simulink library "funcsetup"  (Simulink 5.0)
values from neighbouring files (symbols this model uses):
  RndMeth = 'floor'    [fixpt_interp1.m]
undefined symbols (not defined in the file or in its folder): ErrMax, ErrMax_nonvisible, Nptsmax, Nptsmax_nonvisible, RndMeth_nonvisible, Spacing, Spacing_nonvisible, xData, xData_nonvisible, xDt, xDt_nonvisible, xmax, xMax_nonvisible, xmin, xMin_nonvisible, xScale, xScale_nonvisible, yData, yData_nonvisible, yDt, yDt_nonvisible, yScale, yScale_nonvisible
settings Model: Creator=krishnan  LastModifiedBy=krishnan  ExtModeAutoUpdateStatusClock=off

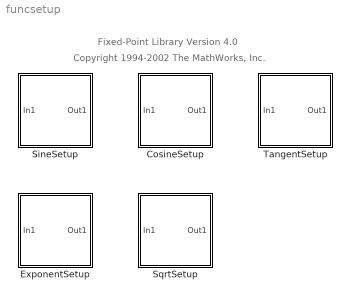
== system funcsetup ==
  note: Fixed-Point Library Version 4.0
  note: Copyright 1994-2002 The MathWorks, Inc.
  CosineSetup : Subsystem  mask(MEGMA CosineSetup){yData=yData, xData=xData, yData_nonvisible=yData_nonvisible, xData_nonvisible=xData_nonvisible, Spacing_nonvisible=Spacing_nonvisible, Nptsmax_nonvisible=Nptsmax_nonvisible, ErrMax_nonvisible=ErrMax_nonvisible, RndMeth_nonvisible=RndMeth_nonvisible, yScale_nonvisible=yScale_nonvisible, yDt_nonvisible=yDt_nonvisible, xScale_nonvisible=xScale_nonvisible, xDt_nonvisible=xDt_nonvisible, xMax_nonvisible=xMax_nonvisible, xMin_nonvisible=xMin_nonvisible, Spacing=Spacing, Nptsmax=Nptsmax, ErrMax=ErrMax, RndMeth=RndMeth, yScale=yScale, xScale=xScale, yDt=yDt, xDt=xDt, xmax=xmax, xmin=xmin}
      mask prompts: Spacing "Allowed spacing 'pow2','even', or 'unrestricted'(default)"; Nptsmax "Maximum number of breakpoints"; ErrMax "Maximum worst case approximation error"; RndMeth "Rounding method 'floor'(default),'ceil','near' or 'zero'"; yScale "Output Scaling"; xScale "Input Scaling"; yDt "Output Datatype"; xDt "Input Datatype"; xmax "Maximum input value of interest"; xmin "Minimum input value of interest"
      mask help: MEGMA CosineSetup
      mask init:
      | FuncStr = 'cos(x)';
      |  par = get_param(gcb,'parent');
      | Recompute = get_param(par,'Recompute');
      | if strcmp(Recompute,'Cache across different MATLAB sessions')
      | Recompute = 3;
      | end
      | if Recompute == 3
      |   if ~isequal(Spacing, Spacing_nonvisible) | ~isequal(Nptsmax,Nptsmax_nonvisible) ...
      | 	|~isequal(ErrMax,ErrMax_nonvisible) | ~isequal(xmin,xMin_nonvisible) ...
      | 	| ~isequal(xmax,xMax_nonvisible) | ~isequal(xDt,xDt_nonvisible) | ...
      | 	~isequal(xScale,xScale_nonvisible) | ~isequal(yDt,yDt_nonvisible) | ...
      | 	~isequal(yScale,yScale_nonvisible) | ~isequal(RndMeth,RndMeth_nonvisible) ...
      | 	| ~isequal(xData,xData_nonvisible) | ~isequal(yData,yData_nonvisible)
      |     text_new_Spacing = get_param(par,'Spacing');
      |     text_new_Nptsmax = get_param(par,'Nptsmax');
      |     text_new_ErrMax  = get_param(par,'ErrMax');
      |     text_new_xmin    = get_param(par,'xmin');
      |     text_new_xmax    = get_param(par,'xmax');
      |     text_new_xDt     = get_param(par,'xDt');
      |     text_new_xScale  = get_param(par,'xScale');
      |     text_new_yDt     = get_param(par,'yDt');
      |     text_new_yScale  = get_param(par,'yScale');
      |     text_new_RndMeth = get_param(par,'RndMeth');
      |     set_param(par,'Spacing_nonvisible',text_new_Spacing);
      |     set_param(par,'Nptsmax_nonvisible',text_new_Nptsmax);
      |     set_param(par,'ErrMax_nonvisible',text_new_ErrMax);
      |     set_param(par,'xMin_nonvisible',text_new_xmin);
      |     set_param(par,'xMax_nonvisible',text_new_xmax);
      |     set_param(par,'xDt_nonvisible',text_new_xDt);
      |     set_param(par,'xScale_nonvisible',text_new_xScale);
      |     set_param(par,'yDt_nonvisible',text_new_yDt);
      |     set_param(par,'yScale_nonvisible',text_new_yScale);
      |     set_param(par,'RndMeth_nonvisible',text_new_RndMeth);
      |     [xData,yData]= fixpt_look1_func_approx(FuncStr,xmin,xmax,xDt,xScale,yDt, ...
      | 					   yScale,RndMeth,...
      | 					   ErrMax,Nptsmax,Spacing,Recompute);
      |     set_param(par,'xData',mat2str(xData));
      |     set_param(par,'yData',mat2str(yData));
      |     set_param(par,'xData_nonvisible',mat2str(xData));
      |     set_param(par,'yData_nonvisible',mat2str(yData));
      |   end
      | end
      mask Help: web(fpbhelp('cosinesetup'));
      mask Display:
      | disp('CosineSetup')
      | patch([2 2 10 10 4 4 8 8 4 4 2 ],[2 10 10 8 8 6 6 4 4 2 2 ],[0 0 0],'bottom-right');
  ExponentSetup : Subsystem  mask(MEGMA ExponentSetup){yData=yData, xData=xData, yData_nonvisible=yData_nonvisible, xData_nonvisible=xData_nonvisible, Spacing_nonvisible=Spacing_nonvisible, Nptsmax_nonvisible=Nptsmax_nonvisible, ErrMax_nonvisible=ErrMax_nonvisible, RndMeth_nonvisible=RndMeth_nonvisible, yScale_nonvisible=yScale_nonvisible, yDt_nonvisible=yDt_nonvisible, xScale_nonvisible=xScale_nonvisible, xDt_nonvisible=xDt_nonvisible, xMax_nonvisible=xMax_nonvisible, xMin_nonvisible=xMin_nonvisible, Spacing=Spacing, Nptsmax=Nptsmax, ErrMax=ErrMax, RndMeth=RndMeth, yScale=yScale, xScale=xScale, yDt=yDt, xDt=xDt, xmax=xmax, xmin=xmin}
      mask prompts: Spacing "Allowed spacing 'pow2','even', or 'unrestricted'(default)"; Nptsmax "Maximum number of breakpoints"; ErrMax "Maximum worst case approximation error"; RndMeth "Rounding method 'floor'(default),'ceil','near' or 'zero'"; yScale "Output Scaling"; xScale "Input Scaling"; yDt "Output Datatype"; xDt "Input Datatype"; xmax "Maximum input value of interest"; xmin "Minimum input value of interest"
      mask help: MEGMA ExponentSetup
      mask init:
      | FuncStr = 'exp(x)';
      |  par = get_param(gcb,'parent');
      | Recompute = get_param(par,'Recompute');
      | if strcmp(Recompute,'Cache across different MATLAB sessions')
      | Recompute = 3;
      | end
      | if Recompute == 3
      |   if ~isequal(Spacing, Spacing_nonvisible) | ~isequal(Nptsmax,Nptsmax_nonvisible) ...
      | 	|~isequal(ErrMax,ErrMax_nonvisible) | ~isequal(xmin,xMin_nonvisible) ...
      | 	| ~isequal(xmax,xMax_nonvisible) | ~isequal(xDt,xDt_nonvisible) | ...
      | 	~isequal(xScale,xScale_nonvisible) | ~isequal(yDt,yDt_nonvisible) | ...
      | 	~isequal(yScale,yScale_nonvisible) | ~isequal(RndMeth,RndMeth_nonvisible) ...
      | 	| ~isequal(xData,xData_nonvisible) | ~isequal(yData,yData_nonvisible)
      |     text_new_Spacing = get_param(par,'Spacing');
      |     text_new_Nptsmax = get_param(par,'Nptsmax');
      |     text_new_ErrMax  = get_param(par,'ErrMax');
      |     text_new_xmin    = get_param(par,'xmin');
      |     text_new_xmax    = get_param(par,'xmax');
      |     text_new_xDt     = get_param(par,'xDt');
      |     text_new_xScale  = get_param(par,'xScale');
      |     text_new_yDt     = get_param(par,'yDt');
      |     text_new_yScale  = get_param(par,'yScale');
      |     text_new_RndMeth = get_param(par,'RndMeth');
      |     set_param(par,'Spacing_nonvisible',text_new_Spacing);
      |     set_param(par,'Nptsmax_nonvisible',text_new_Nptsmax);
      |     set_param(par,'ErrMax_nonvisible',text_new_ErrMax);
      |     set_param(par,'xMin_nonvisible',text_new_xmin);
      |     set_param(par,'xMax_nonvisible',text_new_xmax);
      |     set_param(par,'xDt_nonvisible',text_new_xDt);
      |     set_param(par,'xScale_nonvisible',text_new_xScale);
      |     set_param(par,'yDt_nonvisible',text_new_yDt);
      |     set_param(par,'yScale_nonvisible',text_new_yScale);
      |     set_param(par,'RndMeth_nonvisible',text_new_RndMeth);
      |     [xData,yData]= fixpt_look1_func_approx(FuncStr,xmin,xmax,xDt,xScale,yDt, ...
      | 					   yScale,RndMeth,...
      | 					   ErrMax,Nptsmax,Spacing,Recompute);
      |     set_param(par,'xData',mat2str(xData));
      |     set_param(par,'yData',mat2str(yData));
      |     set_param(par,'xData_nonvisible',mat2str(xData));
      |     set_param(par,'yData_nonvisible',mat2str(yData));
      |   end
      | end
      mask Help: web(fpbhelp('exponentsetup'));
      mask Display:
      | disp('ExponentSetup')
      | patch([2 2 10 10 4 4 8 8 4 4 2 ],[2 10 10 8 8 6 6 4 4 2 2 ],[0 0 0],'bottom-right');
  SineSetup : Subsystem  mask(MEGMA SineSetup){yData=yData, xData=xData, yData_nonvisible=yData_nonvisible, xData_nonvisible=xData_nonvisible, Spacing_nonvisible=Spacing_nonvisible, Nptsmax_nonvisible=Nptsmax_nonvisible, ErrMax_nonvisible=ErrMax_nonvisible, RndMeth_nonvisible=RndMeth_nonvisible, yScale_nonvisible=yScale_nonvisible, yDt_nonvisible=yDt_nonvisible, xScale_nonvisible=xScale_nonvisible, xDt_nonvisible=xDt_nonvisible, xMax_nonvisible=xMax_nonvisible, xMin_nonvisible=xMin_nonvisible, Spacing=Spacing, Nptsmax=Nptsmax, ErrMax=ErrMax, RndMeth=RndMeth, yScale=yScale, xScale=xScale, yDt=yDt, xDt=xDt, xmax=xmax, xmin=xmin}
      mask prompts: Spacing "Allowed spacing 'pow2','even', or 'unrestricted'(default)"; Nptsmax "Maximum number of breakpoints"; ErrMax "Maximum worst case approximation error"; RndMeth "Rounding method 'floor'(default),'ceil','near' or 'zero'"; yScale "Output Scaling"; xScale "Input Scaling"; yDt "Output Datatype"; xDt "Input Datatype"; xmax "Maximum input value of interest"; xmin "Minimum input value of interest"
      mask help: MEGMA SineSetup
      mask init:
      | FuncStr = 'sin(x)';
      |  par = get_param(gcb,'parent');
      | Recompute  = get_param(par,'Recompute');
      | if strcmp(Recompute,'Cache across different MATLAB sessions')
      | Recompute = 3;
      | end
      | if Recompute == 3
      |   if ~isequal(Spacing, Spacing_nonvisible) | ~isequal(Nptsmax,Nptsmax_nonvisible) ...
      | 	|~isequal(ErrMax,ErrMax_nonvisible) | ~isequal(xmin,xMin_nonvisible) ...
      | 	| ~isequal(xmax,xMax_nonvisible) | ~isequal(xDt,xDt_nonvisible) | ...
      | 	~isequal(xScale,xScale_nonvisible) | ~isequal(yDt,yDt_nonvisible) | ...
      | 	~isequal(yScale,yScale_nonvisible) | ~isequal(RndMeth,RndMeth_nonvisible) ...
      | 	| ~isequal(xData,xData_nonvisible) | ~isequal(yData,yData_nonvisible)
      |     text_new_Spacing = get_param(par,'Spacing');
      |     text_new_Nptsmax = get_param(par,'Nptsmax');
      |     text_new_ErrMax  = get_param(par,'ErrMax');
      |     text_new_xmin    = get_param(par,'xmin');
      |     text_new_xmax    = get_param(par,'xmax');
      |     text_new_xDt     = get_param(par,'xDt');
      |     text_new_xScale  = get_param(par,'xScale');
      |     text_new_yDt     = get_param(par,'yDt');
      |     text_new_yScale  = get_param(par,'yScale');
      |     text_new_RndMeth = get_param(par,'RndMeth');
      |     set_param(par,'Spacing_nonvisible',text_new_Spacing);
      |     set_param(par,'Nptsmax_nonvisible',text_new_Nptsmax);
      |     set_param(par,'ErrMax_nonvisible',text_new_ErrMax);
      |     set_param(par,'xMin_nonvisible',text_new_xmin);
      |     set_param(par,'xMax_nonvisible',text_new_xmax);
      |     set_param(par,'xDt_nonvisible',text_new_xDt);
      |     set_param(par,'xScale_nonvisible',text_new_xScale);
      |     set_param(par,'yDt_nonvisible',text_new_yDt);
      |     set_param(par,'yScale_nonvisible',text_new_yScale);
      |     set_param(par,'RndMeth_nonvisible',text_new_RndMeth);
      |     [xData,yData]= fixpt_look1_func_approx(FuncStr,xmin,xmax,xDt,xScale,yDt, ...
      | 					   yScale,RndMeth,...
      | 					   ErrMax,Nptsmax,Spacing,Recompute);
      |     set_param(par,'xData',mat2str(xData));
      |     set_param(par,'yData',mat2str(yData));
      |     set_param(par,'xData_nonvisible',mat2str(xData));
      |     set_param(par,'yData_nonvisible',mat2str(yData));
      |   end
      | end
      mask Help: web(fpbhelp('sinesetup'));
      mask Display:
      | disp('SineSetup')
      | patch([2 2 10 10 4 4 8 8 4 4 2 ],[2 10 10 8 8 6 6 4 4 2 2 ],[0 0 0],'bottom-right');
  SqrtSetup : Subsystem  mask(MEGMA SqrtSetup){yData=yData, xData=xData, yData_nonvisible=yData_nonvisible, xData_nonvisible=xData_nonvisible, Spacing_nonvisible=Spacing_nonvisible, Nptsmax_nonvisible=Nptsmax_nonvisible, ErrMax_nonvisible=ErrMax_nonvisible, RndMeth_nonvisible=RndMeth_nonvisible, yScale_nonvisible=yScale_nonvisible, yDt_nonvisible=yDt_nonvisible, xScale_nonvisible=xScale_nonvisible, xDt_nonvisible=xDt_nonvisible, xMax_nonvisible=xMax_nonvisible, xMin_nonvisible=xMin_nonvisible, Spacing=Spacing, Nptsmax=Nptsmax, ErrMax=ErrMax, RndMeth=RndMeth, yScale=yScale, xScale=xScale, yDt=yDt, xDt=xDt, xmax=xmax, xmin=xmin}
      mask prompts: Spacing "Allowed spacing 'pow2','even', or 'unrestricted'(default)"; Nptsmax "Maximum number of breakpoints"; ErrMax "Maximum worst case approximation error"; RndMeth "Rounding method 'floor'(default),'ceil','near' or 'zero'"; yScale "Output Scaling"; xScale "Input Scaling"; yDt "Output Datatype"; xDt "Input Datatype"; xmax "Maximum input value of interest"; xmin "Minimum input value of interest"
      mask help: MEGMA SqrtSetup
      mask init:
      | FuncStr = 'sqrt(x)';
      |  par = get_param(gcb,'parent');
      | Recompute = get_param(par,'Recompute');
      | if strcmp(Recompute,'Cache across different MATLAB sessions')
      | Recompute = 3;
      | end
      | if Recompute == 3
      |   if ~isequal(Spacing, Spacing_nonvisible) | ~isequal(Nptsmax,Nptsmax_nonvisible) ...
      | 	|~isequal(ErrMax,ErrMax_nonvisible) | ~isequal(xmin,xMin_nonvisible) ...
      | 	| ~isequal(xmax,xMax_nonvisible) | ~isequal(xDt,xDt_nonvisible) | ...
      | 	~isequal(xScale,xScale_nonvisible) | ~isequal(yDt,yDt_nonvisible) | ...
      | 	~isequal(yScale,yScale_nonvisible) | ~isequal(RndMeth,RndMeth_nonvisible) ...
      | 	| ~isequal(xData,xData_nonvisible) | ~isequal(yData,yData_nonvisible)
      |     text_new_Spacing = get_param(par,'Spacing');
      |     text_new_Nptsmax = get_param(par,'Nptsmax');
      |     text_new_ErrMax  = get_param(par,'ErrMax');
      |     text_new_xmin    = get_param(par,'xmin');
      |     text_new_xmax    = get_param(par,'xmax');
      |     text_new_xDt     = get_param(par,'xDt');
      |     text_new_xScale  = get_param(par,'xScale');
      |     text_new_yDt     = get_param(par,'yDt');
      |     text_new_yScale  = get_param(par,'yScale');
      |     text_new_RndMeth = get_param(par,'RndMeth');
      |     set_param(par,'Spacing_nonvisible',text_new_Spacing);
      |     set_param(par,'Nptsmax_nonvisible',text_new_Nptsmax);
      |     set_param(par,'ErrMax_nonvisible',text_new_ErrMax);
      |     set_param(par,'xMin_nonvisible',text_new_xmin);
      |     set_param(par,'xMax_nonvisible',text_new_xmax);
      |     set_param(par,'xDt_nonvisible',text_new_xDt);
      |     set_param(par,'xScale_nonvisible',text_new_xScale);
      |     set_param(par,'yDt_nonvisible',text_new_yDt);
      |     set_param(par,'yScale_nonvisible',text_new_yScale);
      |     set_param(par,'RndMeth_nonvisible',text_new_RndMeth);
      |     [xData,yData]= fixpt_look1_func_approx(FuncStr,xmin,xmax,xDt,xScale,yDt, ...
      | 					   yScale,RndMeth,...
      | 					   ErrMax,Nptsmax,Spacing,Recompute);
      |     set_param(par,'xData',mat2str(xData));
      |     set_param(par,'yData',mat2str(yData));
      |     set_param(par,'xData_nonvisible',mat2str(xData));
      |     set_param(par,'yData_nonvisible',mat2str(yData));
      |   end
      | end
      mask Help: web(fpbhelp('sqrtsetup'));
      mask Display:
      | disp('SqrtSetup')
      | patch([2 2 10 10 4 4 8 8 4 4 2 ],[2 10 10 8 8 6 6 4 4 2 2 ],[0 0 0],'bottom-right');
  TangentSetup : Subsystem  mask(MEGMA TangentSetup){yData=yData, xData=xData, yData_nonvisible=yData_nonvisible, xData_nonvisible=xData_nonvisible, Spacing_nonvisible=Spacing_nonvisible, Nptsmax_nonvisible=Nptsmax_nonvisible, ErrMax_nonvisible=ErrMax_nonvisible, RndMeth_nonvisible=RndMeth_nonvisible, yScale_nonvisible=yScale_nonvisible, yDt_nonvisible=yDt_nonvisible, xScale_nonvisible=xScale_nonvisible, xDt_nonvisible=xDt_nonvisible, xMax_nonvisible=xMax_nonvisible, xMin_nonvisible=xMin_nonvisible, Spacing=Spacing, Nptsmax=Nptsmax, ErrMax=ErrMax, RndMeth=RndMeth, yScale=yScale, xScale=xScale, yDt=yDt, xDt=xDt, xmax=xmax, xmin=xmin}
      mask prompts: Spacing "Allowed spacing 'pow2','even', or 'unrestricted'(default)"; Nptsmax "Maximum number of breakpoints"; ErrMax "Maximum worst case approximation error"; RndMeth "Rounding method 'floor'(default),'ceil','near' or 'zero'"; yScale "Output Scaling"; xScale "Input Scaling"; yDt "Output Datatype"; xDt "Input Datatype"; xmax "Maximum input value of interest"; xmin "Minimum input value of interest"
      mask help: MEGMA TangentSetup
      mask init:
      | FuncStr = 'tan(x)';
      |  par = get_param(gcb,'parent');
      | Recompute = get_param(par,'Recompute');
      | if strcmp(Recompute,'Cache across different MATLAB sessions')
      | Recompute = 3;
      | end
      | if Recompute == 3
      |   if ~isequal(Spacing, Spacing_nonvisible) | ~isequal(Nptsmax,Nptsmax_nonvisible) ...
      | 	|~isequal(ErrMax,ErrMax_nonvisible) | ~isequal(xmin,xMin_nonvisible) ...
      | 	| ~isequal(xmax,xMax_nonvisible) | ~isequal(xDt,xDt_nonvisible) | ...
      | 	~isequal(xScale,xScale_nonvisible) | ~isequal(yDt,yDt_nonvisible) | ...
      | 	~isequal(yScale,yScale_nonvisible) | ~isequal(RndMeth,RndMeth_nonvisible) ...
      | 	| ~isequal(xData,xData_nonvisible) | ~isequal(yData,yData_nonvisible)
      |     text_new_Spacing = get_param(par,'Spacing');
      |     text_new_Nptsmax = get_param(par,'Nptsmax');
      |     text_new_ErrMax  = get_param(par,'ErrMax');
      |     text_new_xmin    = get_param(par,'xmin');
      |     text_new_xmax    = get_param(par,'xmax');
      |     text_new_xDt     = get_param(par,'xDt');
      |     text_new_xScale  = get_param(par,'xScale');
      |     text_new_yDt     = get_param(par,'yDt');
      |     text_new_yScale  = get_param(par,'yScale');
      |     text_new_RndMeth = get_param(par,'RndMeth');
      |     set_param(par,'Spacing_nonvisible',text_new_Spacing);
      |     set_param(par,'Nptsmax_nonvisible',text_new_Nptsmax);
      |     set_param(par,'ErrMax_nonvisible',text_new_ErrMax);
      |     set_param(par,'xMin_nonvisible',text_new_xmin);
      |     set_param(par,'xMax_nonvisible',text_new_xmax);
      |     set_param(par,'xDt_nonvisible',text_new_xDt);
      |     set_param(par,'xScale_nonvisible',text_new_xScale);
      |     set_param(par,'yDt_nonvisible',text_new_yDt);
      |     set_param(par,'yScale_nonvisible',text_new_yScale);
      |     set_param(par,'RndMeth_nonvisible',text_new_RndMeth);
      |     [xData,yData]= fixpt_look1_func_approx(FuncStr,xmin,xmax,xDt,xScale,yDt, ...
      | 					   yScale,RndMeth,...
      | 					   ErrMax,Nptsmax,Spacing,Recompute);
      |     set_param(par,'xData',mat2str(xData));
      |     set_param(par,'yData',mat2str(yData));
      |     set_param(par,'xData_nonvisible',mat2str(xData));
      |     set_param(par,'yData_nonvisible',mat2str(yData));
      |   end
      | end
      mask Help: web(fpbhelp('tangentsetup'));
      mask Display:
      | disp('TangentSetup')
      | patch([2 2 10 10 4 4 8 8 4 4 2 ],[2 10 10 8 8 6 6 4 4 2 2 ],[0 0 0],'bottom-right');

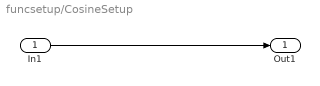
== system funcsetup/CosineSetup ==
  In1 : Inport
  Out1 : Outport
  wires:
  In1/1 -> Out1/1

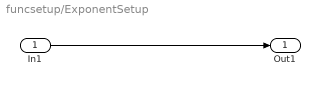
== system funcsetup/ExponentSetup ==
  In1 : Inport
  Out1 : Outport
  wires:
  In1/1 -> Out1/1

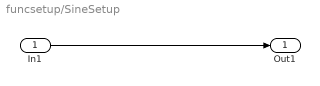
== system funcsetup/SineSetup ==
  In1 : Inport
  Out1 : Outport
  wires:
  In1/1 -> Out1/1

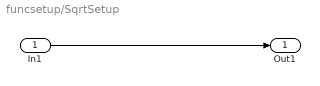
== system funcsetup/SqrtSetup ==
  In1 : Inport
  Out1 : Outport
  wires:
  In1/1 -> Out1/1

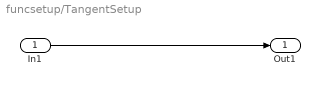
== system funcsetup/TangentSetup ==
  In1 : Inport
  Out1 : Outport
  wires:
  In1/1 -> Out1/1
